simulink model "DRISHTI_Integrated_Telemedicine_System"  (R2026a)
settings: Solver=FixedStepDiscrete  StopTime=1  FixedStep=1
undefined symbols (not defined in the file or in its folder): DRISHTI_aiProcessingSeconds, DRISHTI_aiUnits, DRISHTI_bandwidthMbps, DRISHTI_gradeInput, DRISHTI_imageSizeMB, DRISHTI_modelScore, DRISHTI_patientsPerHour, DRISHTI_qualityScore, DRISHTI_referableRate, DRISHTI_reviewers, DRISHTI_reviewSeconds
settings Model: Creator=SHIVANYA SALES  LastModifiedBy=SHIVANYA SALES

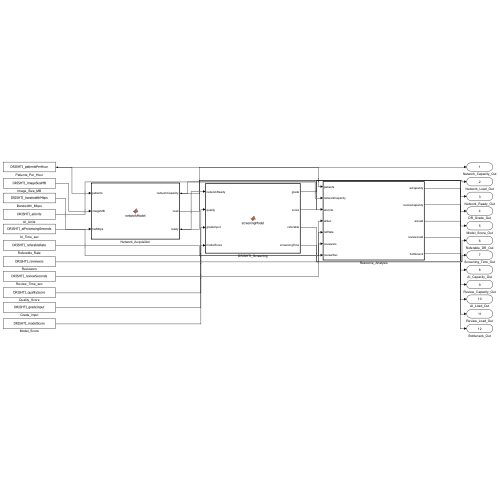
[thumbnail: Simulink's stored preview of the top-level diagram]
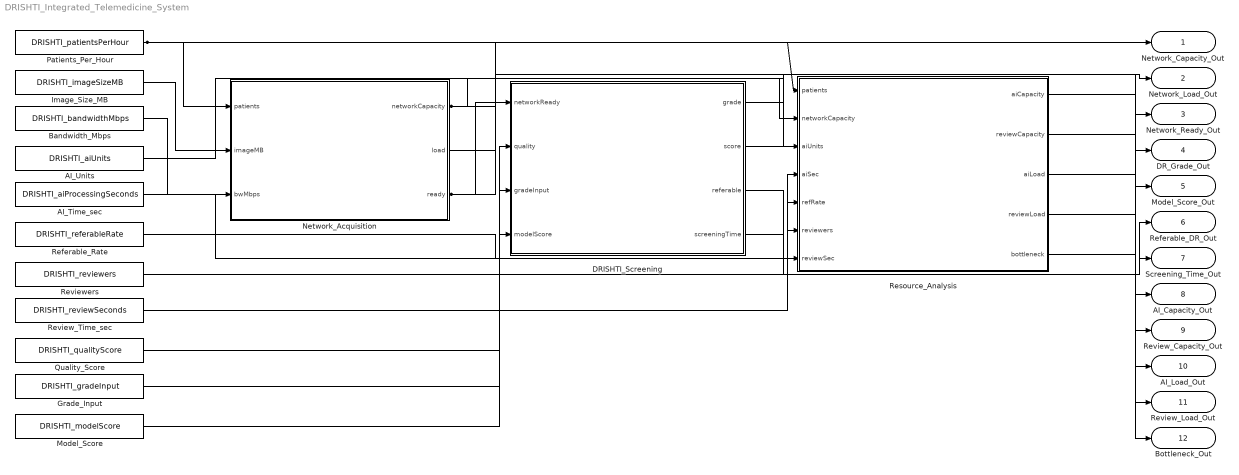
== system DRISHTI_Integrated_Telemedicine_System ==
  AI_Time_sec : Constant  Value=DRISHTI_aiProcessingSeconds
  AI_Units : Constant  Value=DRISHTI_aiUnits
  Bandwidth_Mbps : Constant  Value=DRISHTI_bandwidthMbps
  DRISHTI_Screening : MATLAB Function  TreatAsAtomicUnit=on
  Grade_Input : Constant  Value=DRISHTI_gradeInput
  Image_Size_MB : Constant  Value=DRISHTI_imageSizeMB
  Model_Score : Constant  Value=DRISHTI_modelScore
  Network_Acquisition : MATLAB Function  TreatAsAtomicUnit=on
  Patients_Per_Hour : Constant  Value=DRISHTI_patientsPerHour
  Quality_Score : Constant  Value=DRISHTI_qualityScore
  Referable_Rate : Constant  Value=DRISHTI_referableRate
  Resource_Analysis : MATLAB Function  TreatAsAtomicUnit=on
  Review_Time_sec : Constant  Value=DRISHTI_reviewSeconds
  Reviewers : Constant  Value=DRISHTI_reviewers
  Network_Capacity_Out : Outport
  Network_Load_Out : Outport  Port=2
  Network_Ready_Out : Outport  Port=3
  DR_Grade_Out : Outport  Port=4
  Model_Score_Out : Outport  Port=5
  Referable_DR_Out : Outport  Port=6
  Screening_Time_Out : Outport  Port=7
  AI_Capacity_Out : Outport  Port=8
  Review_Capacity_Out : Outport  Port=9
  AI_Load_Out : Outport  Port=10
  Review_Load_Out : Outport  Port=11
  Bottleneck_Out : Outport  Port=12
  wires:
  Patients_Per_Hour/1 -> Network_Acquisition/1(patients), Resource_Analysis/1(patients)
  Image_Size_MB/1 -> Network_Acquisition/2(imageMB)
  Bandwidth_Mbps/1 -> Network_Acquisition/3(bwMbps)
  Network_Acquisition/3(ready) -> DRISHTI_Screening/1(networkReady), Network_Ready_Out/1
  Quality_Score/1 -> DRISHTI_Screening/2(quality)
  Grade_Input/1 -> DRISHTI_Screening/3(gradeInput)
  Model_Score/1 -> DRISHTI_Screening/4(modelScore)
  Network_Acquisition/1(networkCapacity) -> Resource_Analysis/2(networkCapacity), Network_Capacity_Out/1
  AI_Units/1 -> Resource_Analysis/3(aiUnits)
  AI_Time_sec/1 -> Resource_Analysis/4(aiSec)
  Referable_Rate/1 -> Resource_Analysis/5(refRate)
  Reviewers/1 -> Resource_Analysis/6(reviewers)
  Review_Time_sec/1 -> Resource_Analysis/7(reviewSec)
  Network_Acquisition/2(load) -> Network_Load_Out/1
  DRISHTI_Screening/1(grade) -> DR_Grade_Out/1
  DRISHTI_Screening/2(score) -> Model_Score_Out/1
  DRISHTI_Screening/3(referable) -> Referable_DR_Out/1
  DRISHTI_Screening/4(screeningTime) -> Screening_Time_Out/1
  Resource_Analysis/1(aiCapacity) -> AI_Capacity_Out/1
  Resource_Analysis/2(reviewCapacity) -> Review_Capacity_Out/1
  Resource_Analysis/3(aiLoad) -> AI_Load_Out/1
  Resource_Analysis/4(reviewLoad) -> Review_Load_Out/1
  Resource_Analysis/5(bottleneck) -> Bottleneck_Out/1

== matlab function DRISHTI_Integrated_Telemedicine_System/DRISHTI_Screening ==
  data: networkReady input; grade output; quality input; gradeInput input; modelScore input; score output; referable output; screeningTime output
function [grade,score,referable,screeningTime] = screeningModel(networkReady,quality,gradeInput,modelScore)
grade = -1;
score = 0;
referable = 0;
screeningTime = 0;

if networkReady == 0
    return;
end

if quality < 0.40
    return;
end

grade = gradeInput;
score = modelScore;
screeningTime = 2.4;

if grade >= 2
    referable = 1;
end
end

== matlab function DRISHTI_Integrated_Telemedicine_System/Network_Acquisition ==
  data: patients input; networkCapacity output; imageMB input; bwMbps input; load output; ready output
function [networkCapacity,load,ready] = networkModel(patients,imageMB,bwMbps)
networkCapacity = (bwMbps*3600)/(8*imageMB);
load = patients;
ready = double(load <= networkCapacity);
end

== matlab function DRISHTI_Integrated_Telemedicine_System/Resource_Analysis ==
  data: patients input; aiCapacity output; networkCapacity input; aiUnits input; aiSec input; refRate input; reviewers input; reviewSec input; reviewCapacity output; aiLoad output; reviewLoad output; bottleneck output
function [aiCapacity,reviewCapacity,aiLoad,reviewLoad,bottleneck] = resourceModel(patients,networkCapacity,aiUnits,aiSec,refRate,reviewers,reviewSec)
aiCapacity = aiUnits*(3600/aiSec);
reviewCapacity = reviewers*(3600/reviewSec);

aiLoad = min(patients,networkCapacity);
reviewLoad = aiLoad*refRate;

bottleneck = 0;

if patients > networkCapacity
    bottleneck = 1;
elseif aiLoad > aiCapacity
    bottleneck = 2;
elseif reviewLoad > reviewCapacity
    bottleneck = 3;
end
end
